simulink model "Dist_Models_Integrator"  (R2025b)
settings: Solver=VariableStepAuto  StartTime=0.0  StopTime=10.0  RelTol=1e-3
undefined symbols (not defined in the file or in its folder): DiscIntNeverNeededParam, x0
settings Model: DataDictionary=Model_Vars.sldd  Creator=andrew  LastModifiedBy=andrew

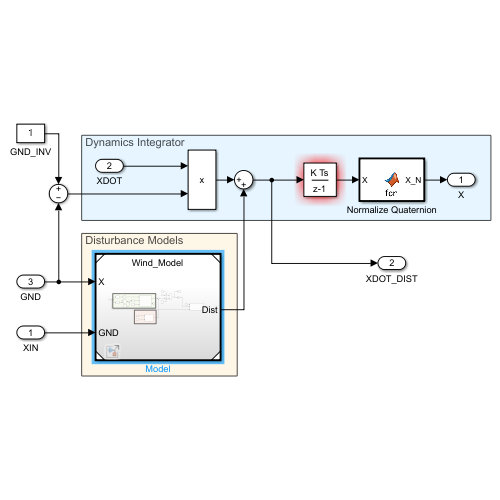
[thumbnail: Simulink's stored preview of the top-level diagram]
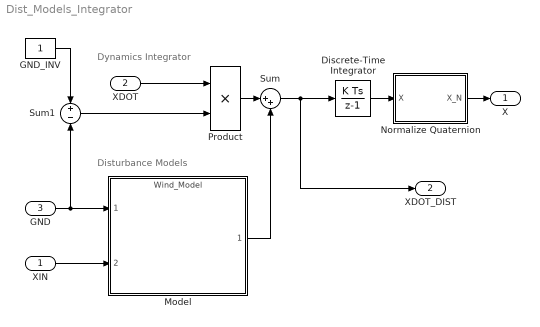
== system Dist_Models_Integrator ==
  note: Dynamics Integrator
  note: Disturbance Models
  XIN : Inport
  XDOT : Inport  Port=2
  GND : Inport  Port=3
  Discrete-Time Integrator : DiscreteIntegrator  InitialCondition=x0  SampleTime=-1  ICPrevOutput=DiscIntNeverNeededParam  ICPrevScaledInput=DiscIntNeverNeededParam
  GND_INV : Constant
  Model : ModelReference  ModelNameDialog=Wind_Model.slx  SimulationMode=Normal  ModelReferenceVersion=1.2
  Normalize Quaternion : MATLAB Function  TreatAsAtomicUnit=on
  Product : Product
  Sum : Sum  Inputs=|++
  Sum1 : Sum  Inputs=+|-
  X : Outport
  XDOT_DIST : Outport  Port=2
  wires:
  Sum/1 -> Discrete-Time Integrator/1, XDOT_DIST/1
  GND/1 -> Model/1, Sum1/2
  GND_INV/1 -> Sum1/1
  Sum1/1 -> Product/2
  Normalize Quaternion/1(X_N) -> X/1
  Product/1 -> Sum/1
  XDOT/1 -> Product/1
  Discrete-Time Integrator/1 -> Normalize Quaternion/1(X)
  XIN/1 -> Model/2
  Model/1 -> Sum/2

== matlab function Dist_Models_Integrator/Normalize Quaternion ==
  data: X input; X_N output
function X_N = fcn(X)
X_N = [X(1:4) / norm(X(1:4)); X(5:end)];
